simulink model "ft_controller_observer"  (R2020b)
settings: Solver=VariableStepAuto  StartTime=0.0  StopTime=10.0  RelTol=1e-3
settings Model: Creator=petir  LastModifiedBy=petir

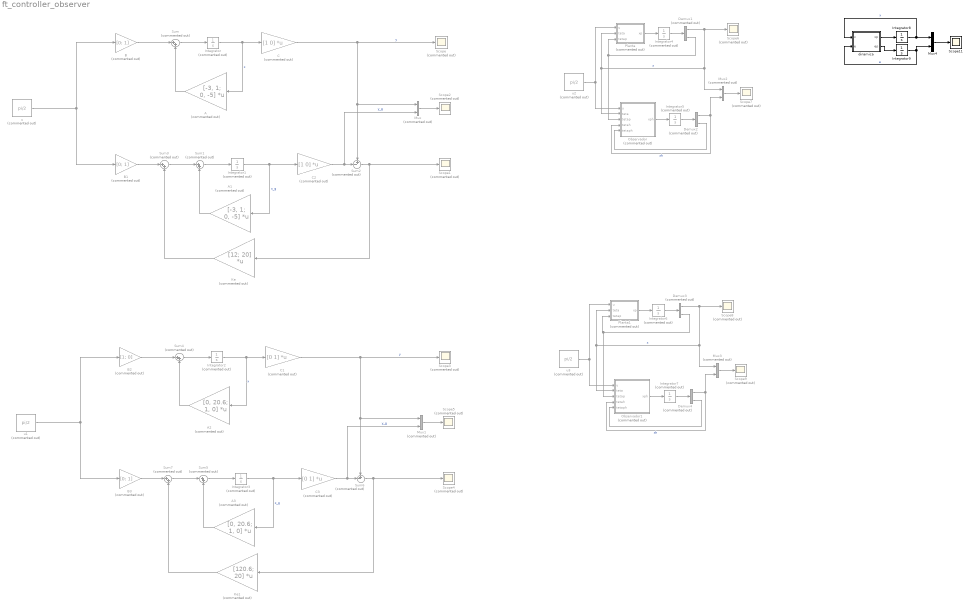
== system ft_controller_observer ==
  A : Gain  Commented=on  Gain=[-3, 1; 0, -5]  Multiplication=Matrix(K*u)
  A1 : Gain  Commented=on  Gain=[-3, 1; 0, -5]  Multiplication=Matrix(K*u)
  A2 : Gain  Commented=on  Gain=[0, 20.6; 1, 0]  Multiplication=Matrix(K*u)
  A3 : Gain  Commented=on  Gain=[0, 20.6; 1, 0]  Multiplication=Matrix(K*u)
  B : Gain  Commented=on  Gain=[0; 1]
  B1 : Gain  Commented=on  Gain=[0; 1]
  B2 : Gain  Commented=on  Gain=[1; 0]
  B3 : Gain  Commented=on  Gain=[0; 1]
  C : Gain  Commented=on  Gain=[1 0]  Multiplication=Matrix(K*u) (u vector)
  C1 : Gain  Commented=on  Gain=[0 1]  Multiplication=Matrix(K*u) (u vector)
  C2 : Gain  Commented=on  Gain=[1 0]  Multiplication=Matrix(K*u) (u vector)
  C3 : Gain  Commented=on  Gain=[0 1]  Multiplication=Matrix(K*u) (u vector)
  Demux{1..4} (4 alike) : Demux  Commented=on  Outputs=2
  Integrator : Integrator  Commented=on  InitialCondition=[1; 0]
  Integrator{1,3,5,7} (4 alike) : Integrator  Commented=on
  Integrator2 : Integrator  Commented=on  InitialCondition=[1; 0]
  Integrator4 : Integrator  Commented=on  InitialCondition=[0; 0]
  Integrator6 : Integrator  Commented=on  InitialCondition=[1; 0]
  Integrator8 : Integrator  InitialCondition=[1; 0]
  Integrator9 : Integrator  InitialCondition=[0.5; 0]
  Ke : Gain  Commented=on  Gain=[12; 20]  Multiplication=Matrix(K*u)
  Ke1 : Gain  Commented=on  Gain=[120.6; 20]  Multiplication=Matrix(K*u)
  Mux{,1..3} (4 alike) : Mux  Commented=on  Inputs=2
  Mux4 : Mux  Inputs=2
  Observador : MATLAB Function  Commented=on  TreatAsAtomicUnit=on
  Observador1 : MATLAB Function  Commented=on  TreatAsAtomicUnit=on
  Planta : MATLAB Function  Commented=on  TreatAsAtomicUnit=on
  Planta1 : MATLAB Function  Commented=on  TreatAsAtomicUnit=on
  Scope{,1..9} (10 alike) : Scope  Commented=on
  Scope11 : Scope
  Sum{,1,3..5,7} (6 alike) : Sum  Commented=on  Inputs=|++
  Sum2 : Sum  Commented=on  Inputs=+-|
  Sum6 : Sum  Commented=on  Inputs=+-|
  dinamica : MATLAB Function  TreatAsAtomicUnit=on
  u{,1..3} (4 alike) : Constant  Commented=on  Value=pi/2  VectorParams1D=off
  wires:
  u/1 -> B1/1, B/1
  B/1 -> Sum/1
  Sum/1 -> Integrator/1
  A/1 -> Sum/2
  Integrator/1 -> C/1, A/1  "x"
  C/1 -> Mux/1, Sum2/1, Scope/1  "y"
  Integrator1/1 -> C2/1, A1/1  "x_g"
  A1/1 -> Sum1/2
  Sum1/1 -> Integrator1/1
  C2/1 -> Mux/2, Sum2/2  "y_g"
  Sum2/1 -> Scope1/1, Ke/1
  Ke/1 -> Sum3/2
  Sum3/1 -> Sum1/1
  B1/1 -> Sum3/1
  Mux/1 -> Scope2/1
  Sum5/1 -> Integrator3/1
  A3/1 -> Sum5/2
  Sum6/1 -> Scope4/1, Ke1/1
  Sum7/1 -> Sum5/1
  Ke1/1 -> Sum7/2
  Integrator3/1 -> C3/1, A3/1  "x_g"
  C1/1 -> Mux1/1, Sum6/1, Scope3/1  "y"
  C3/1 -> Mux1/2, Sum6/2  "y_g"
  Integrator2/1 -> C1/1, A2/1  "x"
  A2/1 -> Sum4/2
  Sum4/1 -> Integrator2/1
  B3/1 -> Sum7/1
  B2/1 -> Sum4/1
  u1/1 -> B3/1, B2/1
  Mux1/1 -> Scope5/1
  Integrator4/1 -> Demux1/1
  Planta/1(xp) -> Integrator4/1
  Demux1/2 -> Observador/3(tetap), Planta/3(tetap)
  Demux1/1 -> Scope6/1, Mux2/1, Observador/2(teta), Planta/2(teta)  "x"
  u2/1 -> Observador/1(u), Planta/1(u)
  Observador/1(xph) -> Integrator5/1
  Integrator5/1 -> Demux2/1
  Demux2/2 -> Observador/5(tetaph)
  Demux2/1 -> Mux2/2, Observador/4(tetah)  "xh"
  Mux2/1 -> Scope7/1
  Observador1/1(xph) -> Integrator7/1
  Demux3/2 -> Observador1/3(tetap), Planta1/3(tetap)
  Integrator6/1 -> Demux3/1
  Demux3/1 -> Scope8/1, Mux3/1, Observador1/2(teta), Planta1/2(teta)  "x"
  Demux4/2 -> Observador1/5(tetaph)
  Demux4/1 -> Mux3/2, Observador1/4(tetah)  "xh"
  Planta1/1(xp) -> Integrator6/1
  Integrator7/1 -> Demux4/1
  Mux3/1 -> Scope9/1
  u3/1 -> Observador1/1(u), Planta1/1(u)
  dinamica/1(xp) -> Integrator8/1
  dinamica/2(ep) -> Integrator9/1
  Integrator8/1 -> Mux4/1, dinamica/1(x)  "x"
  Integrator9/1 -> dinamica/2(e), Mux4/2  "e"
  Mux4/1 -> Scope11/1

== matlab function ft_controller_observer/Observador ==
  data: u input; xph output; teta input; tetap input; tetah input; tetaph input
function xph = fcn(u, teta, tetap, tetah, tetaph)
A = [-3.1, 1; 0, -4.8];
B = [0; 1];
C = [1, 0];
K = [12; 20];

% Observador
xh = [tetah; tetaph];
x = [teta; tetap];

y = C * x;
yh = C *xh;
xph = A * xh + B * u + K *(y - yh);

== matlab function ft_controller_observer/Planta ==
  data: u input; xp output; teta input; tetap input
function xp = fcn(u, teta, tetap)

A = [-3, 1; 0, -5];
B = [0; 1];

% Planta
x = [teta; tetap];
xp = A*x + B*u;

== matlab function ft_controller_observer/Observador1 ==
  data: u input; xph output; teta input; tetap input; tetah input; tetaph input
function xph = fcn(u, teta, tetap, tetah, tetaph)
A = [0, 20.6; 1, 0];
B = [0; 1];
C = [0 1];
K = [120.6; 20];

% Observador
xh = [tetah; tetaph];
x = [teta; tetap];

y = C * x;
yh = C *xh;
xph = A * xh + B * u + K * (y - yh);

== matlab function ft_controller_observer/Planta1 ==
  data: u input; xp output; teta input; tetap input
function xp = fcn(u, teta, tetap)

A = [0, 20.6; 1, 0];
B = [0; 1];

% Planta
x = [teta; tetap];
xp = A*x + B*u;

== matlab function ft_controller_observer/dinamica ==
  data: x input; xp output; e input; ep output
function [xp, ep] = fcn(x, e)

A = [0, 1; 20.6, 0];
B = [0; 1];
C = [1, 0];

% Ganancias
K =[29.6 3.6];
Ke = [16; 84.6];

% Planta
xp = (A-B*K) * x + (B*K)* e;
ep = 0 * x + (A - Ke * C) * e;

% [xp, ep] = [A-B*K, B*K; 0, A - Ke * C];
